simulink model "clase1011"  (R2021a)
settings: Solver=VariableStepAuto  StartTime=0.0  StopTime=10.0  RelTol=1e-3
settings Model: Creator=Santiago  LastModifiedBy=Santiago

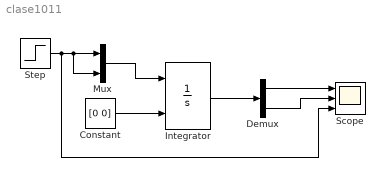
== system clase1011 ==
  Constant : Constant  Value=[0 0]
  Demux : Demux  Outputs=2
  Integrator : Integrator  InitialConditionSource=external
  Mux : Mux  Inputs=2
  Scope : Scope  NumInputPorts=3
  Step : Step  SampleTime=0
  wires:
  Constant/1 -> Integrator/2
  Step/1 -> Scope/3, Mux/2, Mux/1
  Mux/1 -> Integrator/1
  Integrator/1 -> Demux/1
  Demux/1 -> Scope/1
  Demux/2 -> Scope/2
